simulink model "ej2"  (R2013a)
settings: Solver=ode45  StartTime=0.0  StopTime=(N-1)/Fs  MaxStep=1/Fs  MinStep=1/Fs  RelTol=1/Fs  AbsTol=1/Fs
values from neighbouring files (symbols this model uses):
  Fs = 8000    [script1.m]
settings Model: Creator=nazaretrogue  LastModifiedBy=nazaretrogue
settings SolverCC: InitialStep=1/Fs

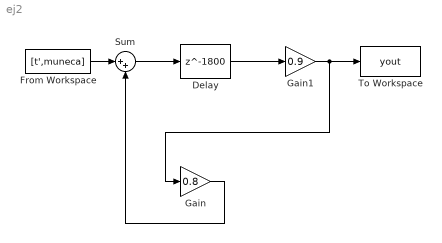
== system ej2 ==
  Delay : Delay  DelayLength=1800  SampleTime=1/Fs
  From Workspace : FromWorkspace  VariableName=[t',muneca]  SampleTime=0
  Gain : Gain  Gain=0.8
  Gain1 : Gain  Gain=0.9
  Sum : Sum  Inputs=|++
  To Workspace : ToWorkspace  VariableName=yout  SampleTime=-1
      settings: MaxDataPoints=N
  wires:
  Sum/1 -> Delay/1
  Delay/1 -> Gain1/1
  Gain1/1 -> Gain/1, To Workspace/1
  Gain/1 -> Sum/2
  From Workspace/1 -> Sum/1
